simulink model "test_diff_IK_trajectories_Succfeetthenbody"  (R2022b)
settings: Solver=ode45  StartTime=0.0  StopTime=2  MaxStep=Step_Time  RelTol=1e-3
InitFcn:
  | O = taskspace_traj(0);
  | p_i = O(1:18);
  | 
  | q_j = IK_geo(p_i);
  | q_i = [p_i(1:6); q_j];
values from neighbouring files (symbols this model uses):
  L_b = 527/1000    (= 0.527)    [quad_properties.m]
  L_h = [53.26 61.84 0.1]/1000    [quad_properties.m]
  L_sh_f = [0 0 280.67]/1000    [quad_properties.m]
  L_sh_h = [0 0 190.62]/1000    [quad_properties.m]
  L_th_f = [0 0 246.5]/1000    [quad_properties.m]
  L_th_h = [0 0 201]/1000    [quad_properties.m]
  L_th_h_mid = [0 0 246.5]/1000    [quad_properties.m]
  W_b = 245.81/1000    (= 0.24581)    [quad_properties.m]
(part 1 of 3)
settings Model: LastModifiedBy=stefa
settings DataIOCC: SaveFormat=Array  ReturnWorkspaceOutputs=off
settings OptimizationCC: BlockReduction=off  BooleanDataType=off
settings DebuggingCC: SaveWithParameterizedLinksMsg=none  UnderspecifiedInitializationDetection=Classic  MergeDetectMultiDrivingBlocksExec=none  SignalResolutionControl=TryResolveAllWithWarning
settings HardwareCC: TargetUnknown=on
settings ModelReferenceCC: PropagateSignalLabelsOutOfModel=off

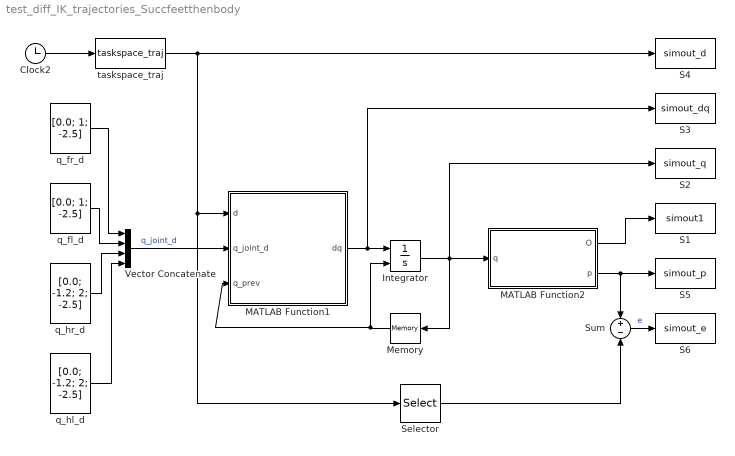
== system test_diff_IK_trajectories_Succfeetthenbody ==
  Clock2 : Clock
  Integrator : Integrator  InitialConditionSource=external
  MATLAB Function1 : MATLAB Function  TreatAsAtomicUnit=on
  MATLAB Function2 : MATLAB Function  TreatAsAtomicUnit=on
  Memory : Memory  InitialCondition=q_i  InheritSampleTime=on
  S1 : ToWorkspace  VariableName=simout1  SaveFormat=Structure With Time  SampleTime=-1
  S2 : ToWorkspace  VariableName=simout_q  SaveFormat=Structure With Time  SampleTime=-1
  S3 : ToWorkspace  VariableName=simout_dq  SaveFormat=Structure With Time  SampleTime=-1
  S4 : ToWorkspace  VariableName=simout_d  SaveFormat=Structure With Time  SampleTime=-1
  S5 : ToWorkspace  VariableName=simout_p  SaveFormat=Structure With Time  SampleTime=-1
  S6 : ToWorkspace  VariableName=simout_e  SaveFormat=Structure With Time  SampleTime=-1
  Selector : Selector  InputPortWidth=54  IndexOptions=Starting index (dialog)  Indices=1  OutputSizes=18
  Sum : Sum  Inputs=+|-
  Vector Concatenate : Concatenate  NumInputs=4
  q_fl_d : Constant  Value=[0.0; 1; -2.5]  VectorParams1D=off
  q_fr_d : Constant  Value=[0.0; 1; -2.5]  VectorParams1D=off
  q_hl_d : Constant  Value=[0.0; -1.2; 2; -2.5]  VectorParams1D=off
  q_hr_d : Constant  Value=[0.0; -1.2; 2; -2.5]  VectorParams1D=off
  taskspace_traj : MATLABFcn  MATLABFcn=taskspace_traj
  wires:
  Clock2/1 -> taskspace_traj/1
  MATLAB Function2/1(O) -> S1/1
  MATLAB Function1/1(dq) -> S3/1, Integrator/1
  Integrator/1 -> S2/1, MATLAB Function2/1(q), Memory/1
  taskspace_traj/1 -> S4/1, MATLAB Function1/1(d), Selector/1
  Memory/1 -> Integrator/2, MATLAB Function1/3(q_prev)
  MATLAB Function2/2(p) -> Sum/1, S5/1
  Sum/1 -> S6/1  "e"
  Selector/1 -> Sum/2
  q_fr_d/1 -> Vector Concatenate/1
  q_fl_d/1 -> Vector Concatenate/2
  q_hr_d/1 -> Vector Concatenate/3
  q_hl_d/1 -> Vector Concatenate/4
  Vector Concatenate/1 -> MATLAB Function1/2(q_joint_d)  "q_joint_d"
